simulink model "bldc_example"  (R2021a)
settings: Solver=FixedStepDiscrete  StartTime=0.0  StopTime=2  RelTol=1e-3  EnableMultiTasking=on
PreLoadFcn:
  | Ts=2e-6;
libraries: AC7DriveInternalModels x2, spsStairGeneratorLib x2, spsThreePhaseSourceLib x1, electricdrivelib x1, spspowerguiLib x1
settings Model: ExtModeAutoUpdateStatusClock=off  Creator=The MathWorks, Inc.  LastModifiedBy=enes_
settings SolverCC: AlgebraicLoopSolver=TrustRegion
settings DataIOCC: LimitDataPoints=on  SaveFormat=Array  ReturnWorkspaceOutputs=off  SignalLoggingName=sigsOut
settings OptimizationCC: ExpressionDepthLimit=2147483647  InitFltsAndDblsToZero=on  LifeSpan=inf
settings DebuggingCC: UnderspecifiedInitializationDetection=Classic  MergeDetectMultiDrivingBlocksExec=none  CheckExecutionContextPreStartOutputMsg=on  SignalResolutionControl=TryResolveAllWithWarning  MultiTaskDSMMsg=warning  MultiTaskCondExecSysMsg=none  FcnCallInpInsideContextMsg=warning  UnconnectedLineMsg=none  StateNameClashWarn=warning  SFUnexpectedBacktrackingDiag=warning  SFNoUnconditionalDefaultTransitionDiag=warning  SFExecutionAtInitializationDiag=none  SFMachineParentedDataDiag=warning  ArithmeticOperatorsInVariantConditions=warning
settings HardwareCC: ProdBitPerPointer=32  ProdBitPerSizeT=32  ProdBitPerPtrDiffT=32  ProdLargestAtomicFloat=None  ProdIntDivRoundTo=Undefined  ProdEndianess=Unspecified  ProdWordSize=32  ProdHWDeviceType=32-bit Generic  TargetUnknown=on
settings ModelReferenceCC: PropagateSignalLabelsOutOfModel=off
settings SFSimCC: SimUseLocalCustomCode=off  CustomCodeUndefinedFunction=UseInterfaceOnly
settings RTWCC: RTWUseLocalCustomCode=off
settings CodeAppCC: StateflowObjectComments=on
settings GRTTargetCC: TargetLangStandard=C89/C90 (ANSI)  CombineOutputUpdateFcns=off  GRTInterface=on
settings ConfigComp: CovMetricSettings=dw  CovSaveCumulativeToWorkspaceVar=on  CovSaveSingleToWorkspaceVar=on  CovExternalEMLEnable=off  CovSFcnEnable=off
settings SimscapeCC: SimscapeNormalizeSystem=off

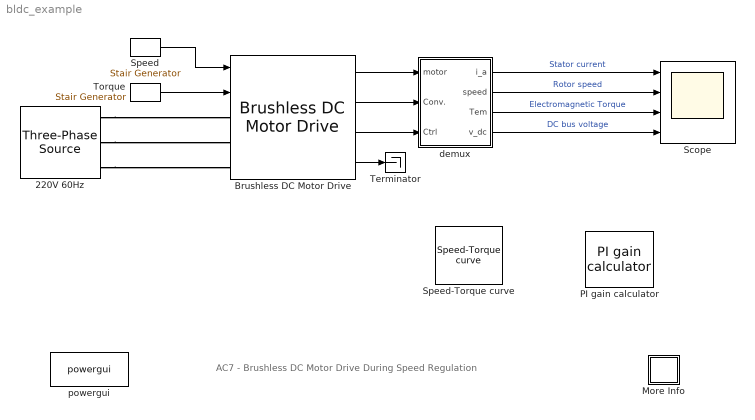
== system bldc_example ==
  note: AC7 - Brushless DC Motor Drive During Speed Regulation
  220V 60Hz : spsThreePhaseSourceLib/Three-Phase Source  InternalConnection=Yg  VoltagePhases=off  Voltage=220  PhaseAngle=0  Voltage_phases=[25e3 25e3 25e3]/sqrt(3)  PhaseAngles_phases=[0 -120 +120]  Frequency=60  NonIdealSource=on  SpecifyImpedance=off  Resistance=0.02  Inductance=0.05e-3  ShortCircuitLevel=100e6  BaseVoltage=25e3  XRratio=7  BusType=swing  Pref=0  Qref=0  Prefabc=[10e3, 10e3, 10e3]  Qrefabc=[0, 0, 0]  Qmin=-inf  Qmax=inf
  Brushless DC Motor Drive : electricdrivelib/AC drives/Brushless DC Motor Drive  Rs=0.2  Lls=8.5e-3  Flat=120  MachineConstant=Flux linkage established by magnets (V.s)  FluxCst=0.175  VoltageCst=146.6077  TorqueCst=1.4  ia=0  ib=0  J=0.089  Friction=0.005  p=4  wm=0  thetam=0  Rsnb_rec=10e3  Csnb_rec=20e-9  Ron_rec=1e-3  Vf_rec=1.3  cap_bus=2000e-6  Rbrake=8  fbrake=4000  activationVoltage=320  shutdownVoltage=310  deviceType=IGBT / Diodes  Ron_inv=1e-3  Vf_inv=0.8  Vfd_inv=0.8  Tf=1e-6  Tt=2e-6  Tf_GTO=10e-6  Tt_GTO=20e-6  Rsnb_inv=5000  Csnb_inv=inf  regulationType=Speed regulation  Acc=1000  Dec=-1000  kp_sc=3.3  ki_sc=300  fc_sc=285  Tsc=140e-6  Tmin=-17.8  Tmax=17.8  h=0.01  freq_max=20e3  Tvect=20e-6  zeta=0.99  Trd=0.13/5  K1=3000  K2=-49500  baseSampleTime=2e-06  outputBusMode=Multiple output buses  busLabels=off  sensorless=off  MechanicalLoad=Torque Tm  modelDetailLevel=Detailed  driveType=AC7  AverageValue=off
      settings: SourceProductBaseCode=PS
  More Info : Subsystem
      settings: OpenFcn=showdemo(bdroot(gcb))
      mask Display: disp('?')
  PI gain calculator : AC7DriveInternalModels/PI gain calculator  mec=[0.089 0.005 4]  specs=on  ele=[0.2 8.5e-3]  lam=0.175  open_loop=off  zeta=0.99  Trd=0.13/5  check=off
      settings: SourceProductBaseCode=PS
  Scope : Scope  NumInputPorts=4
  Speed : spsStairGeneratorLib/Stair Generator  t=[0 1]  e=[300 0]  Ts=Ts
  Speed-Torque curve : AC7DriveInternalModels/Speed-Torque curve  ele=[0.2 8.5e-3]  Flux=0.175  mec=[0.089 0.005 4]  Vdc=310  Tmax=17.8  accel=1000  check=off
      settings: SourceProductBaseCode=PS
  Terminator : Terminator
  Torque : spsStairGeneratorLib/Stair Generator  t=[0.5 1.5]  e=[11 -11]  Ts=Ts
  demux : Subsystem
  powergui : spspowerguiLib/powergui  SimulationMode=Discrete  SampleTime=Ts  frequency=60  Iterations=50  frequencyindice=60  Pbase=100e6  ErrMax=1e-4  UnitsV=kV  UnitsW=MW  buscounter=0  FunctionMessages=off  echomessages=off  EnableUseOfTLC=off  CurrentSourceSwitches=off  DisableSnubberDevices=off  DisableRonSwitches=off  DisableVfSwitches=off  DisplayEquations=off  AutomaticDiscreteSolvers=off  SolverType=Tustin/Backward Euler (TBE)  Interpol=off  ExternalGateDelay=off  methode=off  Ts=0  x0status=blocks  SPID=off  SwTol=0  HookPort=off  NonlinearTolerance=1e-4  nMaxIteration=100  ContinueOnMaxIteration=off  RestoreLinks=warning  ResistiveCurrentMeasurement=off  Frange=[0:2:500]  Ylog=off  Xlog=on  ShowGrid=off  save=off  variable=ZData  structure=0  ZoomFFT=on  StartTime=0.0  cycles=1  DisplayStyle=1  fundamental=60  FreqAxis=off  MaxFrequency=1000  frequencyindicesteady=1  RmsSteady=1  display=off
  wires:
  Brushless DC Motor Drive/1 -> demux/1(motor)
  Brushless DC Motor Drive/2 -> demux/2(Conv.)
  Brushless DC Motor Drive/3 -> demux/3(Ctrl)
  demux/1(i_a) -> Scope/1  "Stator current"
  demux/2(speed) -> Scope/2  "Rotor speed"
  demux/3(Tem) -> Scope/3  "Electromagnetic Torque"
  demux/4(v_dc) -> Scope/4  "DC bus voltage"
  Speed/1 -> Brushless DC Motor Drive/1
  Torque/1 -> Brushless DC Motor Drive/2
  Brushless DC Motor Drive/4 -> Terminator/1
  connections:
  220V 60Hz/RConn1 -- Brushless DC Motor Drive/LConn1
  220V 60Hz/RConn2 -- Brushless DC Motor Drive/LConn2
  220V 60Hz/RConn3 -- Brushless DC Motor Drive/LConn3

== system bldc_example/More Info ==

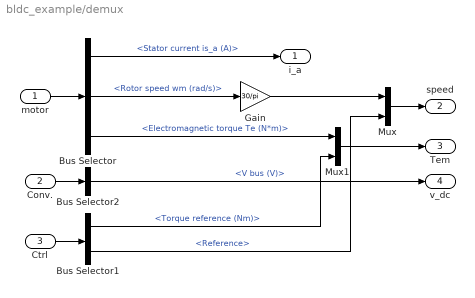
== system bldc_example/demux ==
  motor : Inport
  Conv. : Inport  Port=2
  Ctrl : Inport  Port=3
  Bus Selector : BusSelector  OutputSignals=Stator current is_a (A),Rotor speed wm (rad/s),Electromagnetic torque Te (N*m)
  Bus Selector1 : BusSelector  OutputSignals=Torque reference (Nm),Reference
  Bus Selector2 : BusSelector  OutputSignals=V bus (V)
  Gain : Gain  Gain=30/pi  SaturateOnIntegerOverflow=on  OutDataTypeStr=Inherit: Same as input  ParamDataTypeStr=Inherit: Same as input
  Mux : Mux  Inputs=2
  Mux1 : Mux  Inputs=2
  i_a : Outport  VectorParamsAs1DForOutWhenUnconnected=off
  speed : Outport  Port=2  VectorParamsAs1DForOutWhenUnconnected=off
  Tem : Outport  Port=3  VectorParamsAs1DForOutWhenUnconnected=off
  v_dc : Outport  Port=4  VectorParamsAs1DForOutWhenUnconnected=off
  wires:
  Bus Selector/2 -> Gain/1  "<Rotor speed wm (rad/s)>"
  Bus Selector2/1 -> v_dc/1  "<V bus (V)>"
  Conv./1 -> Bus Selector2/1
  Ctrl/1 -> Bus Selector1/1
  Bus Selector1/1 -> Mux1/2  "<Torque reference (Nm)>"
  Bus Selector1/2 -> Mux/2  "<Reference>"
  Gain/1 -> Mux/1
  Bus Selector/1 -> i_a/1  "<Stator current is_a (A)>"
  Bus Selector/3 -> Mux1/1  "<Electromagnetic torque Te (N*m)>"
  Mux1/1 -> Tem/1
  Mux/1 -> speed/1
  motor/1 -> Bus Selector/1
